simulink model "quadratic"  (R2021a)
settings: Solver=VariableStepAuto  StartTime=0.0  StopTime=10.0  RelTol=1e-3
settings Model: Creator=student  LastModifiedBy=student

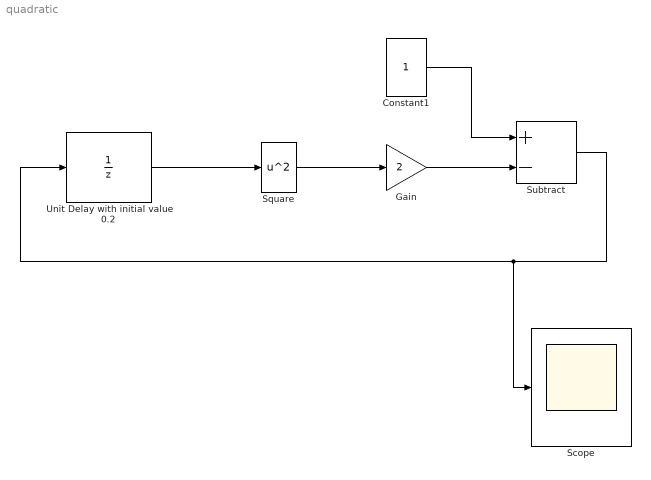
== system quadratic ==
  Constant1 : Constant
  Gain : Gain  Gain=2
  Scope : Scope
  Square : Math  Operator=square  SaturateOnIntegerOverflow=on
  Subtract : Sum  Inputs=+-
  Unit Delay with initial value 0.2 : UnitDelay  InitialCondition=0.2  SampleTime=-1  HasFrameUpgradeWarning=on
  wires:
  Unit Delay with initial value 0.2/1 -> Square/1
  Square/1 -> Gain/1
  Gain/1 -> Subtract/2
  Constant1/1 -> Subtract/1
  Subtract/1 -> Scope/1, Unit Delay with initial value 0.2/1
